simulink subsystem "Main_Kalman_1D_Augmented"  (R2024a)
settings: Solver=VariableStepAuto  StartTime=0.0  StopTime=10.0  RelTol=1e-3
undefined symbols (not defined in the file): Ad_aug, Bd_aug, Q_aug_kf, R_aug_kf
settings Model: Creator=Peter  LastModifiedBy=Peter

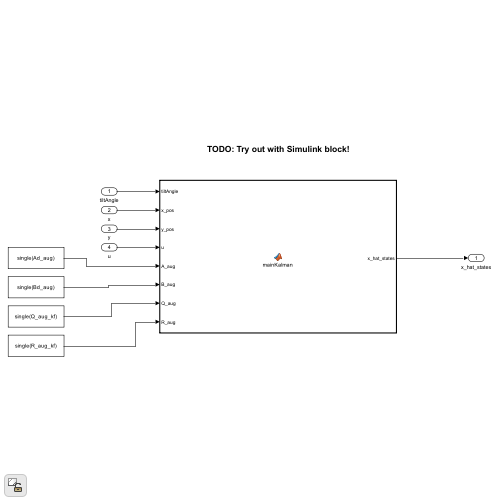
[thumbnail: Simulink's stored preview of the top-level diagram]
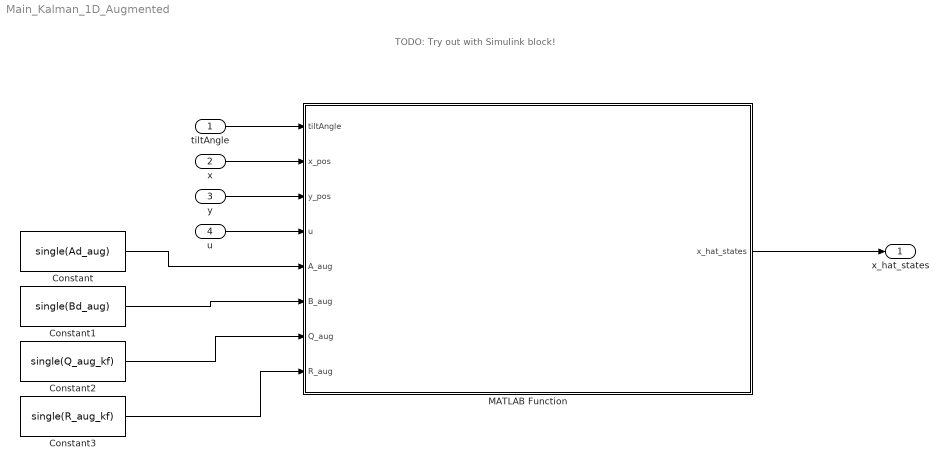
== system Main_Kalman_1D_Augmented ==
  note: TODO: Try out with Simulink block!
  tiltAngle : Inport  OutDataTypeStr=single
  x : Inport  Port=2  OutDataTypeStr=single
  y : Inport  Port=3  OutDataTypeStr=single
  u : Inport  Port=4  OutDataTypeStr=single
  Constant : Constant  Value=single(Ad_aug)  OutDataTypeStr=single
  Constant1 : Constant  Value=single(Bd_aug)  OutDataTypeStr=single
  Constant2 : Constant  Value=single(Q_aug_kf)  OutDataTypeStr=single
  Constant3 : Constant  Value=single(R_aug_kf)  OutDataTypeStr=single
  MATLAB Function : MATLAB Function  TreatAsAtomicUnit=on
  x_hat_states : Outport  OutDataTypeStr=single
  wires:
  y/1 -> MATLAB Function/3(y_pos)
  tiltAngle/1 -> MATLAB Function/1(tiltAngle)
  x/1 -> MATLAB Function/2(x_pos)
  MATLAB Function/1(x_hat_states) -> x_hat_states/1
  Constant1/1 -> MATLAB Function/6(B_aug)
  Constant2/1 -> MATLAB Function/7(Q_aug)
  Constant3/1 -> MATLAB Function/8(R_aug)
  Constant/1 -> MATLAB Function/5(A_aug)
  u/1 -> MATLAB Function/4(u)

== matlab function Main_Kalman_1D_Augmented/MATLAB Function ==
  data: tiltAngle input single; x_hat_states output single; x_pos input single; y_pos input single; u input single; A_aug input single; B_aug input single; Q_aug input single; R_aug input single
function x_hat_states = mainKalman(tiltAngle,x_pos,y_pos,u, A_aug, B_aug, Q_aug, R_aug)
% kalman_filter  Discrete-time Kalman filter for 2-wheeled self-balancing robot
% States: x = [ x; x_dot; theta; theta_dot; i_motor; w_motor]  (6x1)
% Measurements assumed y = [ x_encoder; theta_accel] (2x1)

    A = single(A_aug);
    B = single(B_aug);
    Q = single(Q_aug);
    R = single(R_aug);
    y = single([x_pos;tiltAngle]);
    
    % Dimensions (hard-coded to avoid dynamic size issues)
    nx = 6;   % state dimension
    nz = 2;   % measurement dimension (y size)
    
    persistent xhat P initialized

    if isempty(initialized)
        xhat = zeros(nx,1,'single');
        P    = eye(nx,'single') * single(1e-3);
        initialized = true;
    end
    
        H = single([ 1 0 0 0 0 0;    % x_encoder measures x
                     0 0 1 0 0 0]);   % theta
        
        % Prediction step
        x_pred = A * xhat + B * u;           % 6x1
        P_pred = A * P * A' + Q;             % 6x6
        
        % Update step
        y_pred = H * x_pred;                  % 2x1
        innov = y - y_pred;                   % 2x1
        
        % Innovation covariance S = H*P_pred*H' + R  (2x2)
        S = H * P_pred * H' + R;
        
        % Kalman gain K = P_pred * H' * inv(S)  (4x2)
        S_inv = inv(S);                       % 2x2
        K = P_pred * H' * S_inv;              % 6x2
        
        % State update
        xhat = x_pred + K * innov;            % 6x1
        
        % Joseph stabilized covariance update:
        I = eye(nx,'single');
        P = (I - K*H) * P_pred * (I - K*H)' + K * R * K';
        
        % Outputs
        x_hat_states = xhat;
        %P_out = P;
    
end
